simulink library "simeventsattributes1"  (Simulink 6.6)
undefined symbols (not defined in the file or in its folder): des_support, gcbh
settings Model: Creator=mclune  LastModifiedBy=aapte  ExtModeAutoUpdateStatusClock=off

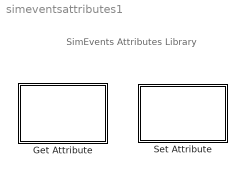
== system simeventsattributes1 ==
  note: SimEvents Attributes Library
  Get Attribute : Subsystem  Priority=1  LoadFcn=des_support('desLoadFcn',gcbh)  StartFcn=des_support('desStartFcn',gcbh)  StopFcn=des_support('desStopFcn',gcbh)  mask(Get Attribute){Attribute1To=Off, Attribute1Name=Attribute1, Attribute1Missing=Error, Attribute1DefaultValue=0, Attribute2To=Off, Attribute2Name=Attribute2, Attribute2Missing=Error, Attribute2DefaultValue=0, Attribute3To=Off, Attribute3Name=Attribute3, Attribute3Missing=Error, Attribute3DefaultValue=0, Attribute4To=Off, Attribute4Name=Attribute4, Attribute4Missing=Error, Attribute4DefaultValue=0, StatNumberDeparted=Off}
      mask prompts: Attribute1To "Send attribute value to signal port A1:"; Attribute1Name "Attribute name:"; Attribute1Missing "Action for missing attribute:"; Attribute1DefaultValue "Default value:"; Attribute2To "Send attribute value to signal port A2:"; Attribute2Name "Attribute name:"; Attribute2Missing "Action for missing attribute:"; Attribute2DefaultValue "Default value:"; Attribute3To "Send attribute value to signal port A3:"; Attribute3Name "Attribute name:"; Attribute3Missing "Action for missing attribute:"; Attribute3DefaultValue "Default value:"; Attribute4To "Send attribute value to signal port A4:"; Attribute4Name "Attribute name:"; Attribute4Missing "Action for missing attribute:"; Attribute4DefaultValue "Default value:"; StatNumberDeparted "Number of entities departed, #d:"
      mask help: Output values of up to four attributes of each entity to signal ports.
      mask init:
      | des_getattributemask(gcb,'init','apply','1');
      settings: CopyFcn=des_support('desCopyFcn',gcbh)  DeleteFcn=des_support('desDeleteFcn',gcbh)  UndoDeleteFcn=des_support('desUndoDeleteFcn',gcbh)  ModelCloseFcn=des_support('desModelCloseFcn',gcbh)  PreSaveFcn=des_support('desPreSaveFcn',gcbh)  PostSaveFcn=des_support('desPostSaveFcn',gcbh)  NameChangeFcn=des_support('desNameChangeFcn',gcbh)  CloseFcn=des_support('desCloseFcn',gcbh)  ErrorFcn=des_error_redirect
      mask Help: helpview(simeventsbhelp)
      mask StyleString: popup(Off|On),edit,popup(Error|Output default value|Output default value and warn),edit,popup(Off|On),edit,popup(Error|Output default value|Output default value and warn),edit,popup(Off|On),edit,popup(Error|Output default value|Output default value and warn),edit,popup(Off|On),edit,popup(Error|Output default value|Output default value and warn),edit,popup(Off|On|Upon stop or pause)
      mask CallbackString: des_getattributemask(gcb,'cbAttributeTo','noapply','1');||des_getattributemask(gcb,'cbAttributeMissing','noapply','1');||des_getattributemask(gcb,'cbAttributeTo','noapply','2');||des_getattributemask(gcb,'cbAttributeMissing','noapply','2');||des_getattributemask(gcb,'cbAttributeTo','noapply','3');||des_getattributemask(gcb,'cbAttributeMissing','noapply','3');||des_getattributemask(gcb,'cbAttributeTo','noapply','4');||des_getattributemask(gcb,'cbAttributeMissing','noapply','4');||des_getattributemask(gcb,'cbStatNumberDeparted','noapply','1');
      mask TabNameString: A1,A1,A1,A1,A2,A2,A2,A2,A3,A3,A3,A3,A4,A4,A4,A4,Statistics
      mask Display:
      | image(des_iconLoad('attrGet.jpg'),'center');
      | port_label('LConn',1,'IN');
      | port_label('RConn',1,'OUT');
  Set Attribute : Subsystem  Priority=1  LoadFcn=des_support('desLoadFcn',gcbh)  StartFcn=des_support('desStartFcn',gcbh)  StopFcn=des_support('desStopFcn',gcbh)  mask(Set Attribute){Attribute1From=Off, Attribute1Name=Attribute1, Attribute1DataType=Double, Attribute1Value=0, Attribute1Create=on, Attribute2From=Off, Attribute2Name=Attribute2, Attribute2DataType=Double, Attribute2Value=0, Attribute2Create=on, Attribute3From=Off, Attribute3Name=Attribute3, Attribute3DataType=Double, Attribute3Value=0, Attribute3Create=on, Attribute4From=Off, Attribute4Name=Attribute4, Attribute4DataType=Double, Attribute4Value=0, Attribute4Create=on, StatNumberDeparted=Off}
      mask prompts: Attribute1From "Attribute assignment:"; Attribute1Name "Attribute name:"; Attribute1DataType "Type:"; Attribute1Value "Value:"; Attribute1Create "Create attribute if not present"; Attribute2From "Attribute assignment:"; Attribute2Name "Attribute name:"; Attribute2DataType "Type:"; Attribute2Value "Value:"; Attribute2Create "Create attribute if not present"; Attribute3From "Attribute assignment:"; Attribute3Name "Attribute name:"; Attribute3DataType "Type:"; Attribute3Value "Value:"; Attribute3Create "Create attribute if not present"; Attribute4From "Attribute assignment:"; Attribute4Name "Attribute name:"; Attribute4DataType "Type:"; Attribute4Value "Value:"; Attribute4Create "Create attribute if not present"; StatNumberDeparted "Number of entities departed, #d:"
      mask help: Set values for up to four attributes of each entity using data from the dialog or signals.
      mask init:
      | des_setattributemask(gcb,'init','apply','1');
      settings: CopyFcn=des_support('desCopyFcn',gcbh)  DeleteFcn=des_support('desDeleteFcn',gcbh)  UndoDeleteFcn=des_support('desUndoDeleteFcn',gcbh)  ModelCloseFcn=des_support('desModelCloseFcn',gcbh)  PreSaveFcn=des_support('desPreSaveFcn',gcbh)  PostSaveFcn=des_support('desPostSaveFcn',gcbh)  NameChangeFcn=des_support('desNameChangeFcn',gcbh)  CloseFcn=des_support('desCloseFcn',gcbh)  ErrorFcn=des_error_redirect
      mask Help: helpview(simeventsbhelp)
      mask StyleString: popup(Off|Specify via dialog|From signal port A1),edit,popup(Double|Integer),edit,checkbox,popup(Off|Specify via dialog|From signal port A2),edit,popup(Double|Integer),edit,checkbox,popup(Off|Specify via dialog|From signal port A3),edit,popup(Double|Integer),edit,checkbox,popup(Off|Specify via dialog|From signal port A4),edit,popup(Double|Integer),edit,checkbox,popup(Off|On|Upon stop or pause)
      mask CallbackString: des_setattributemask(gcb,'cbAttributeFrom','noapply','1');|||||des_setattributemask(gcb,'cbAttributeFrom','noapply','2');|||||des_setattributemask(gcb,'cbAttributeFrom','noapply','3');|||||des_setattributemask(gcb,'cbAttributeFrom','noapply','4');|||||des_setattributemask(gcb,'cbStatNumberDeparted','noapply','1');
      mask TabNameString: A1,A1,A1,A1,A1,A2,A2,A2,A2,A2,A3,A3,A3,A3,A3,A4,A4,A4,A4,A4,Statistics
      mask Display:
      | image(des_iconLoad('attrSet.jpg'),'center');
      | port_label('LConn',1,'IN');
      | port_label('RConn',1,'OUT');

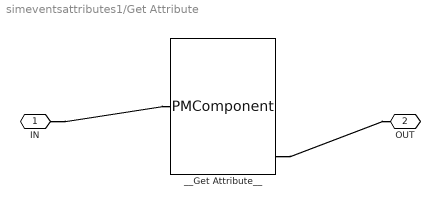
== system simeventsattributes1/Get Attribute ==
  __Get Attribute__ : PMComponent  PhysicalDomain=simevents  SubClassName=DES_GETATTRIBUTE  LeftPortType=desPortIn  RightPortType=desPortOut  LConnTagsString=DI  RConnTagsString=DO|DO|DO|DO|DO|DO
      mask Display:
      | port_label('LConn',1,'IN');
      | port_label('RConn',1,'#d');
      | port_label('RConn',2,'A1');
      | port_label('RConn',3,'A2');
      | port_label('RConn',4,'A3');
      | port_label('RConn',5,'A4');
      | port_label('RConn',6,'OUT');
  IN : PMIOPort  Port=1  Side=Left
  OUT : PMIOPort  Orientation=left  Port=2  Side=Right
  connections:
  IN/RConn1 -- __Get Attribute__/LConn1
  __Get Attribute__/RConn6 -- OUT/RConn1

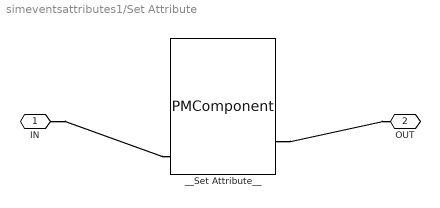
== system simeventsattributes1/Set Attribute ==
  __Set Attribute__ : PMComponent  PhysicalDomain=simevents  SubClassName=DES_SETATTRIBUTE  LeftPortType=desPortIn  RightPortType=desPortOut  LConnTagsString=DI|DI|DI|DI|DI  RConnTagsString=DO|DO
      mask Display:
      | port_label('LConn',1,'A1');
      | port_label('LConn',2,'A2');
      | port_label('LConn',3,'A3');
      | port_label('LConn',4,'A4');
      | port_label('LConn',5,'IN');
      | port_label('RConn',1,'#d');
      | port_label('RConn',2,'OUT');
  IN : PMIOPort  Port=1  Side=Left
  OUT : PMIOPort  Orientation=left  Port=2  Side=Right
  connections:
  IN/RConn1 -- __Set Attribute__/LConn5
  __Set Attribute__/RConn2 -- OUT/RConn1
